simulink model "main_simulation"  (R2020a)
settings: Solver=VariableStepAuto  StartTime=0.0  StopTime=10.0  RelTol=1e-3
settings Model: Creator=rolka  LastModifiedBy=rolka

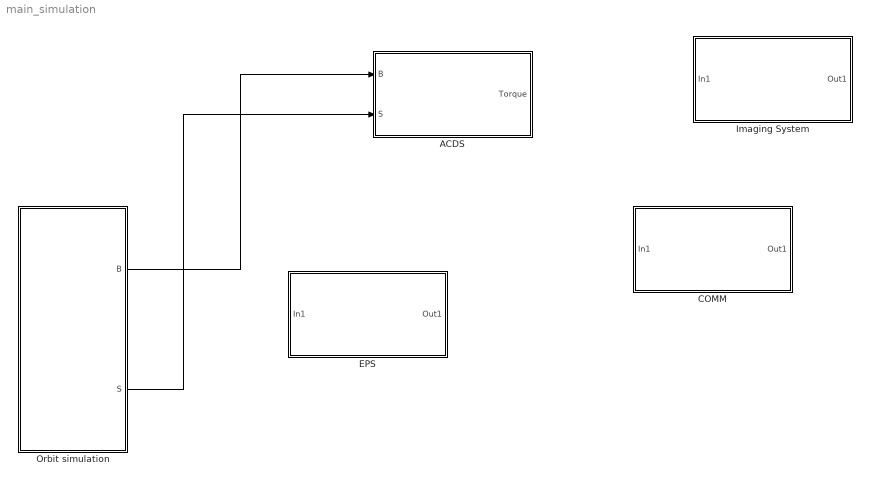
== system main_simulation ==
  ACDS : Subsystem
  COMM : Subsystem
  EPS : Subsystem
  Imaging System : Subsystem
  Orbit simulation : Subsystem
  wires:
  Orbit simulation/1(B) -> ACDS/1(B)
  Orbit simulation/2(S) -> ACDS/2(S)

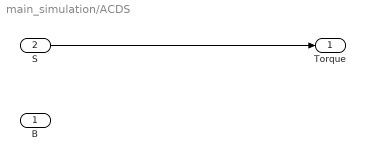
== system main_simulation/ACDS ==
  B : Inport
  S : Inport  Port=2
  Torque : Outport
  wires:
  S/1 -> Torque/1

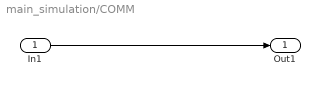
== system main_simulation/COMM ==
  In1 : Inport
  Out1 : Outport
  wires:
  In1/1 -> Out1/1

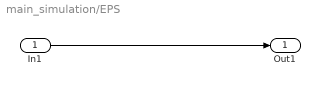
== system main_simulation/EPS ==
  In1 : Inport
  Out1 : Outport
  wires:
  In1/1 -> Out1/1

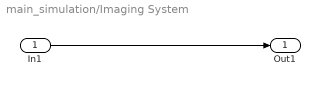
== system main_simulation/Imaging System ==
  In1 : Inport
  Out1 : Outport
  wires:
  In1/1 -> Out1/1

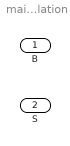
== system main_simulation/Orbit simulation ==
  B : Outport
  S : Outport  Port=2
